simulink model "HumanActionModel"  (R2023a)
settings: Solver=VariableStepAuto  StartTime=0.0  StopTime=5  FixedStep=0.01  RelTol=1e-3
undefined symbols (not defined in the file or in its folder): uD
settings Model: Creator=abane  LastModifiedBy=DELL
settings OptimizationCC: ReuseModelBlockBuffer=off

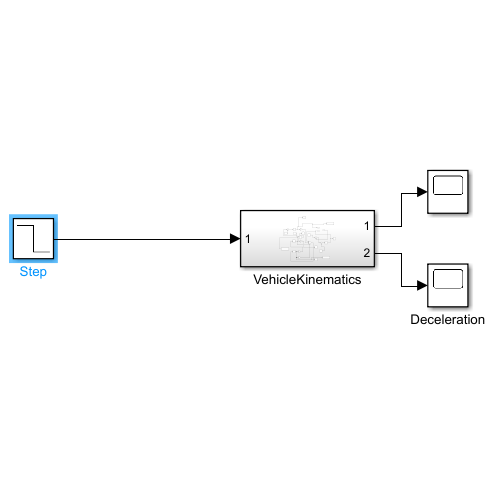
[thumbnail: Simulink's stored preview of the top-level diagram]
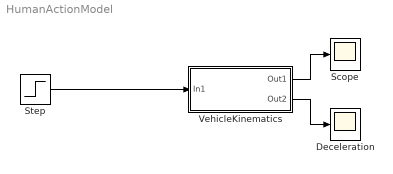
== system HumanActionModel ==
  Deceleration : Scope
  Scope : Scope
  Step : Step  Time=0.04  After=-165  SampleTime=0
  VehicleKinematics : Subsystem
  wires:
  VehicleKinematics/1(Out1) -> Scope/1
  VehicleKinematics/2(Out2) -> Deceleration/1
  Step/1 -> VehicleKinematics/1(In1)

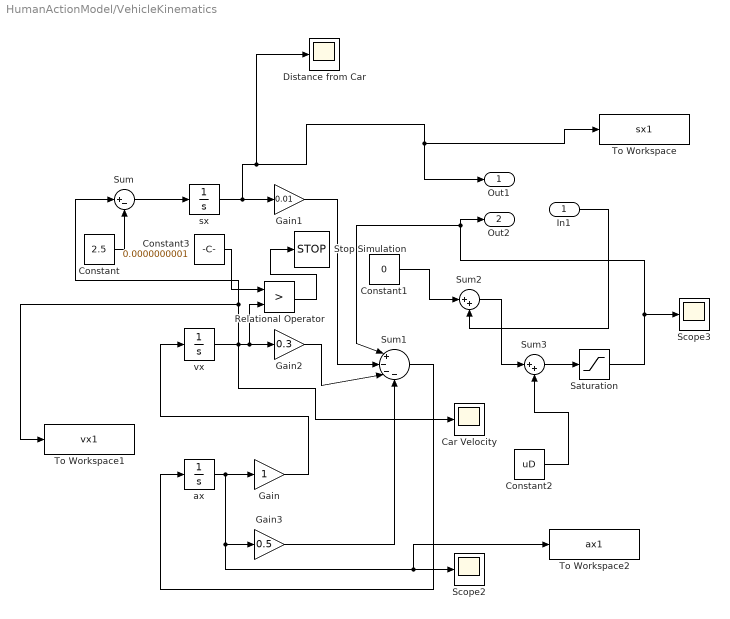
== system HumanActionModel/VehicleKinematics ==
  In1 : Inport
  Car Velocity : Scope
  Constant : Constant  Value=2.5
  Constant1 : Constant  Value=0
  Constant2 : Constant  Value=uD
  Constant3 : Constant  Value=0.0000000001
  Distance from Car : Scope
  Gain : Gain
  Gain1 : Gain  Gain=0.01
  Gain2 : Gain  Gain=0.3
  Gain3 : Gain  Gain=0.5
  Relational Operator : RelationalOperator  Operator=>  OutDataTypeStr=boolean  RndMeth=Simplest  InputSameDT=off
  Saturation : Saturate  UpperLimit=0  LowerLimit=-300
  Scope2 : Scope
  Scope3 : Scope
  Stop Simulation : Stop
  Sum : Sum  Inputs=|+-
  Sum1 : Sum  Inputs=|+---
  Sum2 : Sum  Inputs=|++
  Sum3 : Sum  Inputs=|++
  To Workspace : ToWorkspace  VariableName=sx1  SaveFormat=Timeseries  SampleTime=-1
  To Workspace1 : ToWorkspace  VariableName=vx1  SaveFormat=Timeseries  SampleTime=-1
  To Workspace2 : ToWorkspace  VariableName=ax1  SaveFormat=Timeseries  SampleTime=-1
  ax : Integrator
  sx : Integrator  InitialCondition=-43.8
  vx : Integrator  InitialCondition=41.2
  Out1 : Outport
  Out2 : Outport  Port=2
  wires:
  Constant/1 -> Sum/2
  Sum3/1 -> Saturation/1
  Constant2/1 -> Sum3/2
  Gain1/1 -> Sum1/2
  vx/1 -> Car Velocity/1, To Workspace1/1, Sum/1, Relational Operator/2, Gain2/1
  Saturation/1 -> Out2/1, Sum1/1, Scope3/1
  Gain3/1 -> Sum1/4
  Sum1/1 -> ax/1
  sx/1 -> Distance from Car/1, Out1/1, To Workspace/1, Gain1/1
  Sum2/1 -> Sum3/1
  ax/1 -> To Workspace2/1, Scope2/1, Gain3/1, Gain/1
  In1/1 -> Sum2/2
  Gain2/1 -> Sum1/3
  Constant1/1 -> Sum2/1
  Gain/1 -> vx/1
  Sum/1 -> sx/1
  Relational Operator/1 -> Stop Simulation/1
  Constant3/1 -> Relational Operator/1
